simulink model "CM690A_HwAg0Meas"  (R2013b)
settings: Solver=FixedStepDiscrete  SolverMode=SingleTasking  StartTime=0.0  StopTime=22  FixedStep=0.002  RelTol=1e-3
undefined symbols (not defined in the file): ELECGLBPRM_DEGPERREV_DEGPERREV_F32, ELECGLBPRM_HWAGCENTROFFS_HWDEG_F32, ELECGLBPRM_HWAGSATNLOWRLIM_HWDEG_F32, ELECGLBPRM_HWAGSATNUPPRLIM_HWDEG_F32, ELECGLBPRM_HWAGSCA_ULS_F32, ELECGLBPRM_HWAGSPURGEARRAT_ULS_F32, ELECGLBPRM_HWAGSPURTORINGGEARRATSNSR0_ULS_F32, ELECGLBPRM_HWAGSPURTORINGGEARRATSNSR1_ULS_F32, ELECGLBPRM_NOFLT_CNT_U08, ELECGLBPRM_OFFSTRIMNOTPRFMD_CNT_U08, ELECGLBPRM_PRTCLFLT_CNT_U08, ELECGLBPRM_SKIPSTEPFLT_CNT_U08, ELECGLBPRM_SNSRINTFLT_CNT_U08, ELECGLBPRM_VRNRERRFLT_CNT_U08, FLTINJ_HWAG0MEAS_HWAG0, FLTINJ_HWAG0MEAS_TESTOK, HwAg0IfFlt, HwAg0MeasHwAg0IfFltFailStep, HwAg0MeasHwAg0IfFltPassStep, HwAg0MeasHwAg0Snsr0PrtclFltFailStep, HwAg0MeasHwAg0Snsr0PrtclFltPassStep, HwAg0MeasHwAg0Snsr1PrtclFltFailStep, HwAg0MeasHwAg0Snsr1PrtclFltPassStep, HwAg0MeasSnsr0Rev, HwAg0MeasSnsr1Rev, HwAg0MeasStep, HwAg0MeasVrnrErrThd, HwAg0MfgFlt, HwAg0Snsr0PrtclFlt, HwAg0Snsr1PrtclFlt, HWAG10THTOOTHTRIG_CNT_U08, HWAG11THTOOTHTRIG_CNT_U08, NtcSts1, sigbuilder_block, SigQlfr1
libraries: simulink x30, NxtrNvM x3
(part 3 of 5)

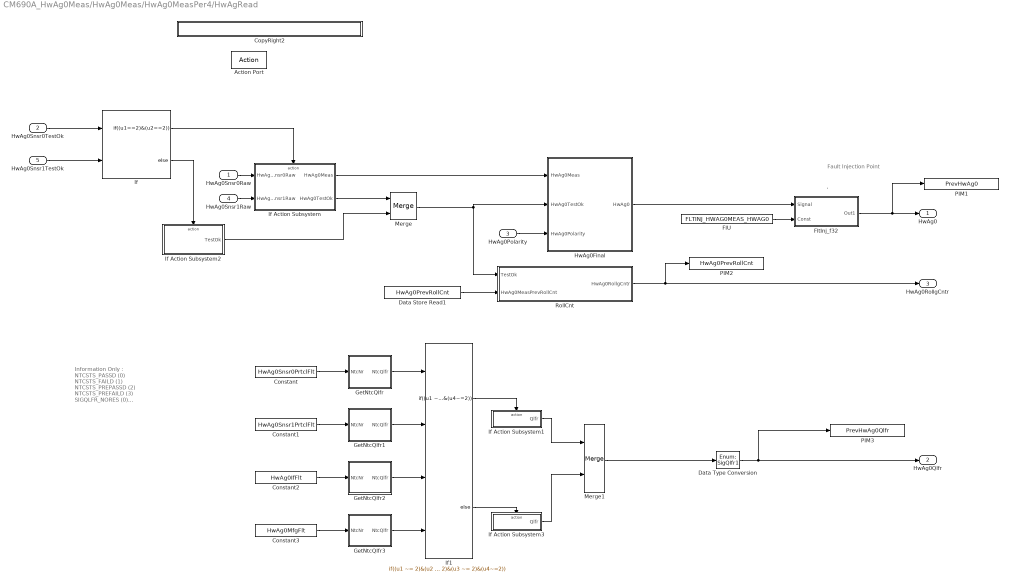
== system CM690A_HwAg0Meas/HwAg0Meas/HwAg0MeasPer4/HwAgRead ==
  note: ,
  note: Fault
      | Injection
      | Point
  note: Information Only :
      |
      | NTCSTS_PASSD            (0)
      | NTCSTS_FAILD              (1)
      | NTCSTS_PREPASSD    (2)
      | NTCSTS_PREFAILD      (3)
      |
      | SIGQLFR_NORES         (0)
      | SIGQLFR_PASSD          (1)
      | SIGQLFR_FAILD            (2)
  HwAg0Snsr0Raw : Inport
  HwAg0Snsr0TestOk : Inport  Port=2
  HwAg0Polarity : Inport  Port=3
  HwAg0Snsr1Raw : Inport  Port=4
  HwAg0Snsr1TestOk : Inport  Port=5
  Action Port : ActionPort  ActionType=then
  Constant : Constant  Value=HwAg0Snsr0PrtclFlt
  Constant1 : Constant  Value=HwAg0Snsr1PrtclFlt
  Constant2 : Constant  Value=HwAg0IfFlt
  Constant3 : Constant  Value=HwAg0MfgFlt
  CopyRight2 : Subsystem  Description=|  mask(Copyright Information){none=on}
      | Copyright info block.                                               
      |                                                                     
      | Place copyright information at the top of every subsystem in design.
      mask prompts: none "No parameters"
      mask help: Place copyright information at the top of every subsystem in design.
      mask Display:
      | NxtrConf = 'Nexteer Confidential';
      | 
      | sys = bdroot; %handle for the current model ("system")
      | first = get_param(sys,'Created');
      | first = first(end-3:end);  %year is last four digits
      | 
      | last = get_param(sys,'LastModifiedDate');
      | if isempty(last)
      |     last = datestr(now,'yyyy');
      | else
      |     last = last(end-3:end);
      | end
      | 
      | if strcmp(first,last)
      |     fprintf('%s -- Copyright %s Nexteer',NxtrConf,first)
      | else
      |     fprintf('%s -- %s%s- %s Nexteer',NxtrConf,char(169),first,last)
      | end
  Data Store Read1 : DataStoreRead  Priority=1  DataStoreName=HwAg0PrevRollCnt
  Data Type Conversion : DataTypeConversion  OutDataTypeStr=Enum: SigQlfr1
  FIU : Constant  Value=FLTINJ_HWAG0MEAS_HWAG0
  FltInj_f32 : Subsystem  RequirementInfo={'linktype_rmi_doors' '0000cf45 (/ESG Group/FDD Module Requirements/EA4 Specific/CM690A_HwAg0Meas)' '#CM690A_108' 'true' 'REQ: CM690A_108' '' } %GIDa_4c7341c4_5f9b_4469_826e_d49718259e6f  TreatAsAtomicUnit=on  VariantControl=FltInj_sim  mask(Fault_Injection){}
      mask help: Fault Injection is a simulation only block for EA4 programs.
  GetNtcQlfr : Subsystem
  GetNtcQlfr1 : Subsystem
  GetNtcQlfr2 : Subsystem
  GetNtcQlfr3 : Subsystem
  HwAg0Final : Subsystem  RequirementInfo={'linktype_rmi_doors' '0000cf45 (/ESG Group/FDD Module Requirements/EA4 Specific/CM690A_HwAg0Meas)' '#CM690A_29' 'true' 'REQ: CM690A_29' '' ; 'linktype_rmi_doors' '0000cf45 (/ESG Group/FDD Module Requirements/EA4 Specific/CM690A_HwAg0Meas)' '#CM690A_32' 'true' 'REQ: CM690A_32' '' ; 'linktype_rmi_doors' '0000cf45 (/ESG Group/FDD Module Requirements/EA4 Specific/CM690A_HwAg0Meas)' '#CM690A_90' 'true' 'REQ: CM690A_90' '' } %GIDa_315d8f1c_91b9_4fec_a381_d34b41dbf245
  If : If  NumInputs=2  IfExpression=(u1==2)&(u2==2)
  If Action Subsystem : Subsystem  TreatAsAtomicUnit=on
  If Action Subsystem1 : Subsystem  TreatAsAtomicUnit=on
  If Action Subsystem2 : Subsystem  TreatAsAtomicUnit=on
  If Action Subsystem3 : Subsystem  TreatAsAtomicUnit=on
  If1 : If  NumInputs=4  IfExpression=(u1 ~= 2)&(u2 ~= 2)&(u3 ~= 2)&(u4~=2)
  Merge : Merge
  Merge1 : Merge
  PIM1 : DataStoreWrite  RequirementInfo={} %GIDa_7b13e776_dea3_4ebd_98b9_3f5e270c50cd  DataStoreName=PrevHwAg0
  PIM2 : DataStoreWrite  RequirementInfo={} %GIDa_14d01694_55be_423b_b81c_a96afe431c02  Priority=2  DataStoreName=HwAg0PrevRollCnt
  PIM3 : DataStoreWrite  RequirementInfo={} %GIDa_a397fdff_e940_40b8_a32d_07bc645247b1  DataStoreName=PrevHwAg0Qlfr
  RollCnt : Stateflow chart  RequirementInfo={} %GIDa_138d63e5_0c8d_44c8_ba68_33eae6500659  TreatAsAtomicUnit=on
  HwAg0 : Outport  RequirementInfo={} %GIDa_98a3716a_95c6_4156_9aa9_7e286709311d
  HwAg0Qlfr : Outport  RequirementInfo={'linktype_rmi_doors' '0000cf45 (/ESG Group/FDD Module Requirements/EA4 Specific/CM690A_HwAg0Meas)' '#CM690A_30' 'true' 'REQ: CM690A_30' '' } %GIDa_8f926389_c076_467c_b7b7_a19e92fafcbc  Port=2
  HwAg0RollgCntr : Outport  RequirementInfo={'linktype_rmi_doors' '0000cf45 (/ESG Group/FDD Module Requirements/EA4 Specific/CM690A_HwAg0Meas)' '#CM690A_31' 'true' 'REQ: CM690A_31' '' } %GIDa_34151e8b_a860_45cc_acf4_67ec6eaad315  Port=3
  wires:
  RollCnt/1(HwAg0RollgCntr) -> PIM2/1, HwAg0RollgCntr/1
  Constant/1 -> GetNtcQlfr/1(NtcNr)
  HwAg0Snsr0TestOk/1 -> If/1
  HwAg0Snsr1TestOk/1 -> If/2
  If/1 -> If Action Subsystem/Action
  If/2 -> If Action Subsystem2/Action
  If Action Subsystem2/1(TestOk) -> Merge/2
  If Action Subsystem/1(HwAg0Meas) -> HwAg0Final/1(HwAg0Meas)
  HwAg0Final/1(HwAg0) -> FltInj_f32/1(Signal)
  Constant1/1 -> GetNtcQlfr1/1(NtcNr)
  Constant2/1 -> GetNtcQlfr2/1(NtcNr)
  GetNtcQlfr/1(NtcQlfr) -> If1/1
  GetNtcQlfr1/1(NtcQlfr) -> If1/2
  GetNtcQlfr2/1(NtcQlfr) -> If1/3
  If1/1 -> If Action Subsystem1/Action
  If1/2 -> If Action Subsystem3/Action
  If Action Subsystem1/1(Qlfr) -> Merge1/1
  If Action Subsystem3/1(Qlfr) -> Merge1/2
  If Action Subsystem/2(HwAg0TestOk) -> Merge/1
  HwAg0Polarity/1 -> HwAg0Final/3(HwAg0Polarity)
  GetNtcQlfr3/1(NtcQlfr) -> If1/4
  Constant3/1 -> GetNtcQlfr3/1(NtcNr)
  FIU/1 -> FltInj_f32/2(Const)
  Merge/1 -> HwAg0Final/2(HwAg0TestOk), RollCnt/1(TestOk)
  FltInj_f32/1(Out1) -> PIM1/1, HwAg0/1
  HwAg0Snsr0Raw/1 -> If Action Subsystem/1(HwAg0Snsr0Raw)
  HwAg0Snsr1Raw/1 -> If Action Subsystem/2(HwAg0Snsr1Raw)
  Data Store Read1/1 -> RollCnt/2(HwAg0MeasPrevRollCnt)
  Merge1/1 -> Data Type Conversion/1
  Data Type Conversion/1 -> PIM3/1, HwAg0Qlfr/1

== system CM690A_HwAg0Meas/HwAg0Meas/HwAg0MeasPer5/CopyRight2 ==

== system CM690A_HwAg0Meas/HwAg0Meas/HwAg0MeasPer5/If Action Subsystem ==
  Action Port : ActionPort  ActionType=then
  CopyRight2 : Subsystem  Description=|  mask(Copyright Information){none=on}
      | Copyright info block.                                               
      |                                                                     
      | Place copyright information at the top of every subsystem in design.
      mask prompts: none "No parameters"
      mask help: Place copyright information at the top of every subsystem in design.
      mask Display:
      | NxtrConf = 'Nexteer Confidential';
      | 
      | sys = bdroot; %handle for the current model ("system")
      | first = get_param(sys,'Created');
      | first = first(end-3:end);  %year is last four digits
      | 
      | last = get_param(sys,'LastModifiedDate');
      | if isempty(last)
      |     last = datestr(now,'yyyy');
      | else
      |     last = last(end-3:end);
      | end
      | 
      | if strcmp(first,last)
      |     fprintf('%s -- Copyright %s Nexteer',NxtrConf,first)
      | else
      |     fprintf('%s -- %s%s- %s Nexteer',NxtrConf,char(169),first,last)
      | end
  Data Type Conversion : DataTypeConversion  OutDataTypeStr=uint8
  NoFlt : Constant  RequirementInfo={} %GIDa_af25b43f_e757_49bd_94aa_be1229c5c8b6  Value=ELECGLBPRM_NOFLT_CNT_U08  OutDataTypeStr=uint8
  NtcSts : simulink/Sources/Enumerated Constant  OutDataTypeStr=Enum: NtcSts1  Value=NtcSts1.NTCSTS_PASSD  SampleTime=inf
  ParamByte : Outport
  TestOk : Outport  Port=2
  wires:
  NtcSts/1 -> Data Type Conversion/1
  NoFlt/1 -> ParamByte/1
  Data Type Conversion/1 -> TestOk/1

== system CM690A_HwAg0Meas/HwAg0Meas/HwAg0MeasPer5/If Action Subsystem1 ==
  Action Port : ActionPort  ActionType=else
  CopyRight2 : Subsystem  Description=|  mask(Copyright Information){none=on}
      | Copyright info block.                                               
      |                                                                     
      | Place copyright information at the top of every subsystem in design.
      mask prompts: none "No parameters"
      mask help: Place copyright information at the top of every subsystem in design.
      mask Display:
      | NxtrConf = 'Nexteer Confidential';
      | 
      | sys = bdroot; %handle for the current model ("system")
      | first = get_param(sys,'Created');
      | first = first(end-3:end);  %year is last four digits
      | 
      | last = get_param(sys,'LastModifiedDate');
      | if isempty(last)
      |     last = datestr(now,'yyyy');
      | else
      |     last = last(end-3:end);
      | end
      | 
      | if strcmp(first,last)
      |     fprintf('%s -- Copyright %s Nexteer',NxtrConf,first)
      | else
      |     fprintf('%s -- %s%s- %s Nexteer',NxtrConf,char(169),first,last)
      | end
  Data Type Conversion : DataTypeConversion  OutDataTypeStr=uint8
  NoFlt : Constant  RequirementInfo={} %GIDa_a79c1974_b7e9_4639_b05c_c7a17ce1d256  Value=ELECGLBPRM_OFFSTRIMNOTPRFMD_CNT_U08  OutDataTypeStr=uint8
  NtcSts : simulink/Sources/Enumerated Constant  OutDataTypeStr=Enum: NtcSts1  Value=NtcSts1.NTCSTS_FAILD  SampleTime=inf
  ParamByte : Outport
  TestOk : Outport  Port=2
  wires:
  NoFlt/1 -> ParamByte/1
  NtcSts/1 -> Data Type Conversion/1
  Data Type Conversion/1 -> TestOk/1

== system CM690A_HwAg0Meas/HwAg0Meas/HwAg0MeasPer5/SetNtcSts ==
  note: Note:
      |
      | - "ISO Fault Debounce Design" Simulink block intent to use here for Simulation purpose only. Do not Code this block
  NtcNr : Inport
  NtcStInfo : Inport  Port=2
  NtcSts : Inport  Port=3
  DebStep : Inport  Port=4
  CopyRight2 : Subsystem  Description=|  mask(Copyright Information){none=on}
      | Copyright info block.                                               
      |                                                                     
      | Place copyright information at the top of every subsystem in design.
      mask prompts: none "No parameters"
      mask help: Place copyright information at the top of every subsystem in design.
      mask Display:
      | NxtrConf = 'Nexteer Confidential';
      | 
      | sys = bdroot; %handle for the current model ("system")
      | first = get_param(sys,'Created');
      | first = first(end-3:end);  %year is last four digits
      | 
      | last = get_param(sys,'LastModifiedDate');
      | if isempty(last)
      |     last = datestr(now,'yyyy');
      | else
      |     last = last(end-3:end);
      | end
      | 
      | if strcmp(first,last)
      |     fprintf('%s -- Copyright %s Nexteer',NxtrConf,first)
      | else
      |     fprintf('%s -- %s%s- %s Nexteer',NxtrConf,char(169),first,last)
      | end
  Data Store Write : DataStoreWrite  DataStoreName=Ntc0X1F9Qlfr
  Ground : Ground
  ISO Fault Debounce Design : Stateflow chart  TreatAsAtomicUnit=on
      settings: AttributesFormatString=|
      | Simulation Purpose Only.
      | Do Not Code this block
      | Diagnostic Manager Owns this requirement
  Scope1 : Scope  NumInputPorts=3
      settings: YMin=-5~-5~-5  YMax=5~5~5  SaveName=ScopeData5
  Terminator : Terminator
  Terminator1 : Terminator
  wires:
  Ground/1 -> ISO Fault Debounce Design/3(SvcClr)
  ISO Fault Debounce Design/1(Qualifier) -> Data Store Write/1, Scope1/3
  DebStep/1 -> Scope1/2, ISO Fault Debounce Design/2(DebStep)
  NtcSts/1 -> Scope1/1, ISO Fault Debounce Design/1(NtcSts)
  NtcNr/1 -> Terminator/1
  NtcStInfo/1 -> Terminator1/1

== system CM690A_HwAg0Meas/HwAg0Meas/HwAg0MeasInit1/GetRefTmr1MicroSec32bit/CopyRight2 ==

== system CM690A_HwAg0Meas/HwAg0Meas/HwAg0MeasInit1/GetTiSpan1MicroSec32bit/CopyRight2 ==

== system CM690A_HwAg0Meas/HwAg0Meas/HwAg0MeasInit1/IoHwAb_SetFctPrphlHwAg0/CopyRight2 ==

== system CM690A_HwAg0Meas/HwAg0Meas/HwAg0MeasPer1/GetRefTmr1MicroSec32bit1/CopyRight2 ==

== system CM690A_HwAg0Meas/HwAg0Meas/HwAg0MeasPer1/GetTiSpan1MicroSec32bit/CopyRight2 ==

== system CM690A_HwAg0Meas/HwAg0Meas/HwAg0MeasPer1/IncrementCount/CopyRight2 ==

== system CM690A_HwAg0Meas/HwAg0Meas/HwAg0MeasPer1/ResetCount/CopyRight2 ==

== system CM690A_HwAg0Meas/HwAg0Meas/HwAg0MeasPer2/Snsr0Read/CopyRight2 ==

== system CM690A_HwAg0Meas/HwAg0Meas/HwAg0MeasPer2/Snsr0Read/DebStepSelection ==
  TestOk : Inport
  CopyRight2 : Subsystem  Description=|  mask(Copyright Information){none=on}
      | Copyright info block.                                               
      |                                                                     
      | Place copyright information at the top of every subsystem in design.
      mask prompts: none "No parameters"
      mask help: Place copyright information at the top of every subsystem in design.
      mask Display:
      | NxtrConf = 'Nexteer Confidential';
      | 
      | sys = bdroot; %handle for the current model ("system")
      | first = get_param(sys,'Created');
      | first = first(end-3:end);  %year is last four digits
      | 
      | last = get_param(sys,'LastModifiedDate');
      | if isempty(last)
      |     last = datestr(now,'yyyy');
      | else
      |     last = last(end-3:end);
      | end
      | 
      | if strcmp(first,last)
      |     fprintf('%s -- Copyright %s Nexteer',NxtrConf,first)
      | else
      |     fprintf('%s -- %s%s- %s Nexteer',NxtrConf,char(169),first,last)
      | end
  NTCFailStepCal : Constant  Value=HwAg0MeasHwAg0Snsr0PrtclFltFailStep
  NTCPassStepCal : Constant  Value=HwAg0MeasHwAg0Snsr0PrtclFltPassStep
  Switch : Switch  Criteria=u2 > Threshold  Threshold=2
  DebStep : Outport  OutDataTypeStr=uint16
  wires:
  NTCFailStepCal/1 -> Switch/1
  Switch/1 -> DebStep/1
  NTCPassStepCal/1 -> Switch/3
  TestOk/1 -> Switch/2

== system CM690A_HwAg0Meas/HwAg0Meas/HwAg0MeasPer2/Snsr0Read/Do nothing ==
  Action Port : ActionPort  ActionType=else
  CopyRight2 : Subsystem  Description=|  mask(Copyright Information){none=on}
      | Copyright info block.                                               
      |                                                                     
      | Place copyright information at the top of every subsystem in design.
      mask prompts: none "No parameters"
      mask help: Place copyright information at the top of every subsystem in design.
      mask Display:
      | NxtrConf = 'Nexteer Confidential';
      | 
      | sys = bdroot; %handle for the current model ("system")
      | first = get_param(sys,'Created');
      | first = first(end-3:end);  %year is last four digits
      | 
      | last = get_param(sys,'LastModifiedDate');
      | if isempty(last)
      |     last = datestr(now,'yyyy');
      | else
      |     last = last(end-3:end);
      | end
      | 
      | if strcmp(first,last)
      |     fprintf('%s -- Copyright %s Nexteer',NxtrConf,first)
      | else
      |     fprintf('%s -- %s%s- %s Nexteer',NxtrConf,char(169),first,last)
      | end

== system CM690A_HwAg0Meas/HwAg0Meas/HwAg0MeasPer2/Snsr0Read/RawHwAgRead ==
  Snsr0CS : Inport
  Snsr0FRS : Inport  Port=2
  Snsr0FCCN : Inport  Port=3
  Snsr0Data : Inport  Port=4
  Snsr0Id : Inport  Port=5
  Bus Selector : BusSelector  OutputSignals=RawHwAg,TestOk,ParamByte
  Bus Selector1 : BusSelector  OutputSignals=RawHwAg,TestOk,ParamByte
  CopyRight2 : Subsystem  Description=|  mask(Copyright Information){none=on}
      | Copyright info block.                                               
      |                                                                     
      | Place copyright information at the top of every subsystem in design.
      mask prompts: none "No parameters"
      mask help: Place copyright information at the top of every subsystem in design.
      mask Display:
      | NxtrConf = 'Nexteer Confidential';
      | 
      | sys = bdroot; %handle for the current model ("system")
      | first = get_param(sys,'Created');
      | first = first(end-3:end);  %year is last four digits
      | 
      | last = get_param(sys,'LastModifiedDate');
      | if isempty(last)
      |     last = datestr(now,'yyyy');
      | else
      |     last = last(end-3:end);
      | end
      | 
      | if strcmp(first,last)
      |     fprintf('%s -- Copyright %s Nexteer',NxtrConf,first)
      | else
      |     fprintf('%s -- %s%s- %s Nexteer',NxtrConf,char(169),first,last)
      | end
  If : If  RequirementInfo={} %GIDa_46781e8b_8ae4_49ab_b4ce_f2a8b4411ed9  IfExpression=u1 ~= 0
  Merge : Merge
  Merge1 : Merge
  Merge2 : Merge
  NewMsg : Subsystem  TreatAsAtomicUnit=on
  NoNewMsg : Subsystem  RequirementInfo={'linktype_rmi_doors' '0000cf45 (/ESG Group/FDD Module Requirements/EA4 Specific/CM690A_HwAg0Meas)' '#CM690A_47' 'true' 'REQ: CM690A_47' '' } %GIDa_ed38ddaf_6377_4824_8afe_3c38153c265e  TreatAsAtomicUnit=on
      mask Display: disp('NoNewMsg')
  RawHwAg : Outport
  TestOk : Outport  Port=2
  ParamByte : Outport  Port=3
  wires:
  Snsr0FRS/1 -> If/1
  If/1 -> NewMsg/Action  "NoFault"
  If/2 -> NoNewMsg/Action  "Fault"
  Snsr0CS/1 -> NewMsg/1(Snsr0CS)
  NewMsg/1(Out1) -> Bus Selector/1
  NoNewMsg/1(Out1) -> Bus Selector1/1
  Bus Selector1/1 -> Merge2/1  "<RawHwAg>"
  Bus Selector/1 -> Merge2/2  "<RawHwAg>"
  Bus Selector1/2 -> Merge/1  "<TestOk>"
  Bus Selector/2 -> Merge/2  "<TestOk>"
  Bus Selector1/3 -> Merge1/1  "<ParamByte>"
  Bus Selector/3 -> Merge1/2  "<ParamByte>"
  Merge2/1 -> RawHwAg/1  "RawHwAg"
  Merge/1 -> TestOk/1  "TestOk"
  Merge1/1 -> ParamByte/1  "ParamByte"
  Snsr0FCCN/1 -> NewMsg/2(Snsr0FCCN)
  Snsr0Data/1 -> NewMsg/4(Snsr0Data)
  Snsr0Id/1 -> NewMsg/3(Snsr0Id)

== system CM690A_HwAg0Meas/HwAg0Meas/HwAg0MeasPer2/Snsr0Read/Read the Flag ==
  RegInpRSENT4FND : Inport
  Action Port : ActionPort  ActionType=then
  CopyRight2 : Subsystem  Description=|  mask(Copyright Information){none=on}
      | Copyright info block.                                               
      |                                                                     
      | Place copyright information at the top of every subsystem in design.
      mask prompts: none "No parameters"
      mask help: Place copyright information at the top of every subsystem in design.
      mask Display:
      | NxtrConf = 'Nexteer Confidential';
      | 
      | sys = bdroot; %handle for the current model ("system")
      | first = get_param(sys,'Created');
      | first = first(end-3:end);  %year is last four digits
      | 
      | last = get_param(sys,'LastModifiedDate');
      | if isempty(last)
      |     last = datestr(now,'yyyy');
      | else
      |     last = last(end-3:end);
      | end
      | 
      | if strcmp(first,last)
      |     fprintf('%s -- Copyright %s Nexteer',NxtrConf,first)
      | else
      |     fprintf('%s -- %s%s- %s Nexteer',NxtrConf,char(169),first,last)
      | end
  RSENT4DummyRead : Terminator
  wires:
  RegInpRSENT4FND/1 -> RSENT4DummyRead/1

== system CM690A_HwAg0Meas/HwAg0Meas/HwAg0MeasPer2/Snsr0Read/SetNtcSts ==
  note: Note:
      |
      | - "ISO Fault Debounce Design" Simulink block intent to use here for Simulation purpose only. Do not Code this block
  NtcNr : Inport
  NtcStInfo : Inport  Port=2
  NtcSts : Inport  Port=3
  DebStep : Inport  Port=4
  CopyRight2 : Subsystem  Description=|  mask(Copyright Information){none=on}
      | Copyright info block.                                               
      |                                                                     
      | Place copyright information at the top of every subsystem in design.
      mask prompts: none "No parameters"
      mask help: Place copyright information at the top of every subsystem in design.
      mask Display:
      | NxtrConf = 'Nexteer Confidential';
      | 
      | sys = bdroot; %handle for the current model ("system")
      | first = get_param(sys,'Created');
      | first = first(end-3:end);  %year is last four digits
      | 
      | last = get_param(sys,'LastModifiedDate');
      | if isempty(last)
      |     last = datestr(now,'yyyy');
      | else
      |     last = last(end-3:end);
      | end
      | 
      | if strcmp(first,last)
      |     fprintf('%s -- Copyright %s Nexteer',NxtrConf,first)
      | else
      |     fprintf('%s -- %s%s- %s Nexteer',NxtrConf,char(169),first,last)
      | end
  Data Store Write : DataStoreWrite  DataStoreName=Ntc0x093Qlfr
  Ground : Ground
  ISO Fault Debounce Design : Stateflow chart  TreatAsAtomicUnit=on
      settings: AttributesFormatString=|
      | Simulation Purpose Only.
      | Do Not Code this block
      | Diagnostic Manager Owns this requirement
  Scope1 : Scope  NumInputPorts=3
      settings: YMin=-5~-5~-5  YMax=5~5~5  SaveName=ScopeData5
  Terminator : Terminator
  Terminator1 : Terminator
  wires:
  Ground/1 -> ISO Fault Debounce Design/3(SvcClr)
  ISO Fault Debounce Design/1(Qualifier) -> Data Store Write/1, Scope1/3
  DebStep/1 -> Scope1/2, ISO Fault Debounce Design/2(DebStep)
  NtcSts/1 -> Scope1/1, ISO Fault Debounce Design/1(NtcSts)
  NtcNr/1 -> Terminator/1
  NtcStInfo/1 -> Terminator1/1

== system CM690A_HwAg0Meas/HwAg0Meas/HwAg0MeasPer2/Snsr0Read1/CopyRight2 ==

== system CM690A_HwAg0Meas/HwAg0Meas/HwAg0MeasPer3/Snsr1Read/CopyRight2 ==

== system CM690A_HwAg0Meas/HwAg0Meas/HwAg0MeasPer3/Snsr1Read/DebStepSelection ==
  TestOk : Inport
  CopyRight2 : Subsystem  Description=|  mask(Copyright Information){none=on}
      | Copyright info block.                                               
      |                                                                     
      | Place copyright information at the top of every subsystem in design.
      mask prompts: none "No parameters"
      mask help: Place copyright information at the top of every subsystem in design.
      mask Display:
      | NxtrConf = 'Nexteer Confidential';
      | 
      | sys = bdroot; %handle for the current model ("system")
      | first = get_param(sys,'Created');
      | first = first(end-3:end);  %year is last four digits
      | 
      | last = get_param(sys,'LastModifiedDate');
      | if isempty(last)
      |     last = datestr(now,'yyyy');
      | else
      |     last = last(end-3:end);
      | end
      | 
      | if strcmp(first,last)
      |     fprintf('%s -- Copyright %s Nexteer',NxtrConf,first)
      | else
      |     fprintf('%s -- %s%s- %s Nexteer',NxtrConf,char(169),first,last)
      | end
  NTCFailStepCal : Constant  Value=HwAg0MeasHwAg0Snsr1PrtclFltFailStep
  NTCPassStepCal : Constant  Value=HwAg0MeasHwAg0Snsr1PrtclFltPassStep
  Switch : Switch  Criteria=u2 > Threshold  Threshold=2
  DebStep : Outport  OutDataTypeStr=uint16
  wires:
  NTCFailStepCal/1 -> Switch/1
  Switch/1 -> DebStep/1
  NTCPassStepCal/1 -> Switch/3
  TestOk/1 -> Switch/2

== system CM690A_HwAg0Meas/HwAg0Meas/HwAg0MeasPer3/Snsr1Read/Do nothing1 ==
  Action Port : ActionPort  ActionType=else
  CopyRight2 : Subsystem  Description=|  mask(Copyright Information){none=on}
      | Copyright info block.                                               
      |                                                                     
      | Place copyright information at the top of every subsystem in design.
      mask prompts: none "No parameters"
      mask help: Place copyright information at the top of every subsystem in design.
      mask Display:
      | NxtrConf = 'Nexteer Confidential';
      | 
      | sys = bdroot; %handle for the current model ("system")
      | first = get_param(sys,'Created');
      | first = first(end-3:end);  %year is last four digits
      | 
      | last = get_param(sys,'LastModifiedDate');
      | if isempty(last)
      |     last = datestr(now,'yyyy');
      | else
      |     last = last(end-3:end);
      | end
      | 
      | if strcmp(first,last)
      |     fprintf('%s -- Copyright %s Nexteer',NxtrConf,first)
      | else
      |     fprintf('%s -- %s%s- %s Nexteer',NxtrConf,char(169),first,last)
      | end

== system CM690A_HwAg0Meas/HwAg0Meas/HwAg0MeasPer3/Snsr1Read/Do nothing2 ==
  Action Port : ActionPort  ActionType=else
  CopyRight2 : Subsystem  Description=|  mask(Copyright Information){none=on}
      | Copyright info block.                                               
      |                                                                     
      | Place copyright information at the top of every subsystem in design.
      mask prompts: none "No parameters"
      mask help: Place copyright information at the top of every subsystem in design.
      mask Display:
      | NxtrConf = 'Nexteer Confidential';
      | 
      | sys = bdroot; %handle for the current model ("system")
      | first = get_param(sys,'Created');
      | first = first(end-3:end);  %year is last four digits
      | 
      | last = get_param(sys,'LastModifiedDate');
      | if isempty(last)
      |     last = datestr(now,'yyyy');
      | else
      |     last = last(end-3:end);
      | end
      | 
      | if strcmp(first,last)
      |     fprintf('%s -- Copyright %s Nexteer',NxtrConf,first)
      | else
      |     fprintf('%s -- %s%s- %s Nexteer',NxtrConf,char(169),first,last)
      | end

== system CM690A_HwAg0Meas/HwAg0Meas/HwAg0MeasPer3/Snsr1Read/RawHwAgRead ==
  Snsr1CS : Inport
  Snsr1FRS : Inport  Port=2
  Snsr1FCCN : Inport  Port=3
  Snsr1Data : Inport  Port=4
  Snsr1Id : Inport  Port=5
  Bus Selector : BusSelector  OutputSignals=RawHwAg,TestOk,ParamByte
  Bus Selector1 : BusSelector  OutputSignals=RawHwAg,TestOk,ParamByte
  CopyRight2 : Subsystem  Description=|  mask(Copyright Information){none=on}
      | Copyright info block.                                               
      |                                                                     
      | Place copyright information at the top of every subsystem in design.
      mask prompts: none "No parameters"
      mask help: Place copyright information at the top of every subsystem in design.
      mask Display:
      | NxtrConf = 'Nexteer Confidential';
      | 
      | sys = bdroot; %handle for the current model ("system")
      | first = get_param(sys,'Created');
      | first = first(end-3:end);  %year is last four digits
      | 
      | last = get_param(sys,'LastModifiedDate');
      | if isempty(last)
      |     last = datestr(now,'yyyy');
      | else
      |     last = last(end-3:end);
      | end
      | 
      | if strcmp(first,last)
      |     fprintf('%s -- Copyright %s Nexteer',NxtrConf,first)
      | else
      |     fprintf('%s -- %s%s- %s Nexteer',NxtrConf,char(169),first,last)
      | end
  If : If  RequirementInfo={} %GIDa_7644cdbb_66a8_49f6_a4d4_60348c8cfce1  IfExpression=u1 ~= 0
  Merge : Merge
  Merge1 : Merge
  Merge2 : Merge
  NewMsg : Subsystem  TreatAsAtomicUnit=on
  NoNewMsg : Subsystem  RequirementInfo={'linktype_rmi_doors' '0000cf45 (/ESG Group/FDD Module Requirements/EA4 Specific/CM690A_HwAg0Meas)' '#CM690A_64' 'true' 'REQ: CM690A_64' '' } %GIDa_10b4e8f5_e554_4d89_a490_9a22ba77e950  TreatAsAtomicUnit=on
      mask Display: disp('NoNewMsg')
  RawHwAg : Outport
  TestOk : Outport  Port=2
  ParamByte : Outport  Port=3
  wires:
  Snsr1FRS/1 -> If/1
  If/1 -> NewMsg/Action  "NoFault"
  If/2 -> NoNewMsg/Action  "Fault"
  Snsr1CS/1 -> NewMsg/1(Snsr1CS)
  NewMsg/1(Out1) -> Bus Selector/1
  NoNewMsg/1(Out1) -> Bus Selector1/1
  Bus Selector1/1 -> Merge2/1  "<RawHwAg>"
  Bus Selector/1 -> Merge2/2  "<RawHwAg>"
  Bus Selector1/2 -> Merge/1  "<TestOk>"
  Bus Selector/2 -> Merge/2  "<TestOk>"
  Bus Selector1/3 -> Merge1/1  "<ParamByte>"
  Bus Selector/3 -> Merge1/2  "<ParamByte>"
  Merge2/1 -> RawHwAg/1  "RawHwAg"
  Merge/1 -> TestOk/1  "TestOk"
  Merge1/1 -> ParamByte/1  "ParamByte"
  Snsr1FCCN/1 -> NewMsg/2(Snsr1FCCN)
  Snsr1Data/1 -> NewMsg/4(Snsr1Data)
  Snsr1Id/1 -> NewMsg/3(Snsr1Id)

== system CM690A_HwAg0Meas/HwAg0Meas/HwAg0MeasPer3/Snsr1Read/Read the Flag ==
  RegInpRSENT4FND : Inport
  Action Port : ActionPort  ActionType=then
  CopyRight2 : Subsystem  Description=|  mask(Copyright Information){none=on}
      | Copyright info block.                                               
      |                                                                     
      | Place copyright information at the top of every subsystem in design.
      mask prompts: none "No parameters"
      mask help: Place copyright information at the top of every subsystem in design.
      mask Display:
      | NxtrConf = 'Nexteer Confidential';
      | 
      | sys = bdroot; %handle for the current model ("system")
      | first = get_param(sys,'Created');
      | first = first(end-3:end);  %year is last four digits
      | 
      | last = get_param(sys,'LastModifiedDate');
      | if isempty(last)
      |     last = datestr(now,'yyyy');
      | else
      |     last = last(end-3:end);
      | end
      | 
      | if strcmp(first,last)
      |     fprintf('%s -- Copyright %s Nexteer',NxtrConf,first)
      | else
      |     fprintf('%s -- %s%s- %s Nexteer',NxtrConf,char(169),first,last)
      | end
  RSENT4DummyRead : Terminator
  wires:
  RegInpRSENT4FND/1 -> RSENT4DummyRead/1

== system CM690A_HwAg0Meas/HwAg0Meas/HwAg0MeasPer3/Snsr1Read/SetNtcSts ==
  note: Note:
      |
      | - "ISO Fault Debounce Design" Simulink block intent to use here for Simulation purpose only. Do not Code this block
  NtcNr : Inport
  NtcStInfo : Inport  Port=2
  NtcSts : Inport  Port=3
  DebStep : Inport  Port=4
  CopyRight2 : Subsystem  Description=|  mask(Copyright Information){none=on}
      | Copyright info block.                                               
      |                                                                     
      | Place copyright information at the top of every subsystem in design.
      mask prompts: none "No parameters"
      mask help: Place copyright information at the top of every subsystem in design.
      mask Display:
      | NxtrConf = 'Nexteer Confidential';
      | 
      | sys = bdroot; %handle for the current model ("system")
      | first = get_param(sys,'Created');
      | first = first(end-3:end);  %year is last four digits
      | 
      | last = get_param(sys,'LastModifiedDate');
      | if isempty(last)
      |     last = datestr(now,'yyyy');
      | else
      |     last = last(end-3:end);
      | end
      | 
      | if strcmp(first,last)
      |     fprintf('%s -- Copyright %s Nexteer',NxtrConf,first)
      | else
      |     fprintf('%s -- %s%s- %s Nexteer',NxtrConf,char(169),first,last)
      | end
  Data Store Write : DataStoreWrite  DataStoreName=Ntc0x095Qlfr
  Ground : Ground
  ISO Fault Debounce Design : Stateflow chart  TreatAsAtomicUnit=on
      settings: AttributesFormatString=|
      | Simulation Purpose Only.
      | Do Not Code this block
      | Diagnostic Manager Owns this requirement
  Scope1 : Scope  NumInputPorts=3
      settings: YMin=-5~-5~-5  YMax=5~5~5  SaveName=ScopeData5
  Terminator : Terminator
  Terminator1 : Terminator
  wires:
  Ground/1 -> ISO Fault Debounce Design/3(SvcClr)
  ISO Fault Debounce Design/1(Qualifier) -> Data Store Write/1, Scope1/3
  DebStep/1 -> Scope1/2, ISO Fault Debounce Design/2(DebStep)
  NtcSts/1 -> Scope1/1, ISO Fault Debounce Design/1(NtcSts)
  NtcNr/1 -> Terminator/1
  NtcStInfo/1 -> Terminator1/1

== system CM690A_HwAg0Meas/HwAg0Meas/HwAg0MeasPer3/Snsr1Read/SyncPulse ==
  note: Information only:
      |
      | - Sensors are synchronized if they receive 104us tick wide SPCT low pulse.
  note: Follow below steps in same order:
      |
      | 1. Send Sensor Synchronization command Pulse (RegOutRSENT4SPCT = 103U)
      | 1a. asm"syncm"
      | 2. NRS Flag Check: If the flag (RegInpRSENT4NRS==1) is Set Clear the flag RegOutRSENT4NRC=1
      | 2a. 2us wait timer
      | 3. Execute RegOutRSENT4SPCT = 103U
  RegInpRSENT4NRS : Inport
  Action Port : ActionPort  ActionType=then
  CopyRight2 : Subsystem  Description=|  mask(Copyright Information){none=on}
      | Copyright info block.                                               
      |                                                                     
      | Place copyright information at the top of every subsystem in design.
      mask prompts: none "No parameters"
      mask help: Place copyright information at the top of every subsystem in design.
      mask Display:
      | NxtrConf = 'Nexteer Confidential';
      | 
      | sys = bdroot; %handle for the current model ("system")
      | first = get_param(sys,'Created');
      | first = first(end-3:end);  %year is last four digits
      | 
      | last = get_param(sys,'LastModifiedDate');
      | if isempty(last)
      |     last = datestr(now,'yyyy');
      | else
      |     last = last(end-3:end);
      | end
      | 
      | if strcmp(first,last)
      |     fprintf('%s -- Copyright %s Nexteer',NxtrConf,first)
      | else
      |     fprintf('%s -- %s%s- %s Nexteer',NxtrConf,char(169),first,last)
      | end
  GetRefTmr1MicroSec32bit : Subsystem
      settings: AttributesFormatString=Client Call : Start Time
  GetTiSpan1MicroSec32bit : Subsystem
  Ground1 : Ground
  Ground2 : Ground
  Terminator : Terminator
  Terminator1 : Terminator
  RegOutRSENT4SPCT : Outport
  RegOutRSENT4NRC : Outport  Port=2
  wires:
  Ground1/1 -> RegOutRSENT4SPCT/1
  Ground2/1 -> RegOutRSENT4NRC/1
  RegInpRSENT4NRS/1 -> Terminator/1
  GetTiSpan1MicroSec32bit/1(TiSpan) -> Terminator1/1
  GetRefTmr1MicroSec32bit/1(RefTmr) -> GetTiSpan1MicroSec32bit/1(RefTmr)

== system CM690A_HwAg0Meas/HwAg0Meas/HwAg0MeasPer3/Snsr1Read1/CopyRight2 ==

== system CM690A_HwAg0Meas/HwAg0Meas/HwAg0MeasPer4/HwAgPrevRead/CopyRight2 ==

== system CM690A_HwAg0Meas/HwAg0Meas/HwAg0MeasPer4/HwAgRead/CopyRight2 ==

== system CM690A_HwAg0Meas/HwAg0Meas/HwAg0MeasPer4/HwAgRead/FltInj_f32 ==
  note: Inport #2 must be constant
      | Const: FltInjectionLocType
  note: EA4.x Fault Injection
  note: This block requires no modification by FDD author.
      |
      | This block does not actually simulate any fault injection.  It is simply a pass-thru.
      |
      | The Const port (#2) simply terminates its signal, but we are trying to force the FDD author
      | to properly use the FltInjectionLocType enumeration in FDD model.
  Signal : Inport
  Const : Inport  Port=2
  Terminator : Terminator
  Out1 : Outport
  wires:
  Const/1 -> Terminator/1
  Signal/1 -> Out1/1

== system CM690A_HwAg0Meas/HwAg0Meas/HwAg0MeasPer4/HwAgRead/GetNtcQlfr ==
  NtcNr : Inport
  CopyRight2 : Subsystem  Description=|  mask(Copyright Information){none=on}
      | Copyright info block.                                               
      |                                                                     
      | Place copyright information at the top of every subsystem in design.
      mask prompts: none "No parameters"
      mask help: Place copyright information at the top of every subsystem in design.
      mask Display:
      | NxtrConf = 'Nexteer Confidential';
      | 
      | sys = bdroot; %handle for the current model ("system")
      | first = get_param(sys,'Created');
      | first = first(end-3:end);  %year is last four digits
      | 
      | last = get_param(sys,'LastModifiedDate');
      | if isempty(last)
      |     last = datestr(now,'yyyy');
      | else
      |     last = last(end-3:end);
      | end
      | 
      | if strcmp(first,last)
      |     fprintf('%s -- Copyright %s Nexteer',NxtrConf,first)
      | else
      |     fprintf('%s -- %s%s- %s Nexteer',NxtrConf,char(169),first,last)
      | end
  Data Store Read : DataStoreRead  DataStoreName=Ntc0x093Qlfr
  Terminator : Terminator
  NtcQlfr : Outport
  wires:
  Data Store Read/1 -> NtcQlfr/1
  NtcNr/1 -> Terminator/1

== system CM690A_HwAg0Meas/HwAg0Meas/HwAg0MeasPer4/HwAgRead/GetNtcQlfr1 ==
  NtcNr : Inport
  CopyRight2 : Subsystem  Description=|  mask(Copyright Information){none=on}
      | Copyright info block.                                               
      |                                                                     
      | Place copyright information at the top of every subsystem in design.
      mask prompts: none "No parameters"
      mask help: Place copyright information at the top of every subsystem in design.
      mask Display:
      | NxtrConf = 'Nexteer Confidential';
      | 
      | sys = bdroot; %handle for the current model ("system")
      | first = get_param(sys,'Created');
      | first = first(end-3:end);  %year is last four digits
      | 
      | last = get_param(sys,'LastModifiedDate');
      | if isempty(last)
      |     last = datestr(now,'yyyy');
      | else
      |     last = last(end-3:end);
      | end
      | 
      | if strcmp(first,last)
      |     fprintf('%s -- Copyright %s Nexteer',NxtrConf,first)
      | else
      |     fprintf('%s -- %s%s- %s Nexteer',NxtrConf,char(169),first,last)
      | end
  Data Store Read : DataStoreRead  DataStoreName=Ntc0x095Qlfr
  Terminator : Terminator
  NtcQlfr : Outport
  wires:
  Data Store Read/1 -> NtcQlfr/1
  NtcNr/1 -> Terminator/1

== system CM690A_HwAg0Meas/HwAg0Meas/HwAg0MeasPer4/HwAgRead/GetNtcQlfr2 ==
  NtcNr : Inport
  CopyRight2 : Subsystem  Description=|  mask(Copyright Information){none=on}
      | Copyright info block.                                               
      |                                                                     
      | Place copyright information at the top of every subsystem in design.
      mask prompts: none "No parameters"
      mask help: Place copyright information at the top of every subsystem in design.
      mask Display:
      | NxtrConf = 'Nexteer Confidential';
      | 
      | sys = bdroot; %handle for the current model ("system")
      | first = get_param(sys,'Created');
      | first = first(end-3:end);  %year is last four digits
      | 
      | last = get_param(sys,'LastModifiedDate');
      | if isempty(last)
      |     last = datestr(now,'yyyy');
      | else
      |     last = last(end-3:end);
      | end
      | 
      | if strcmp(first,last)
      |     fprintf('%s -- Copyright %s Nexteer',NxtrConf,first)
      | else
      |     fprintf('%s -- %s%s- %s Nexteer',NxtrConf,char(169),first,last)
      | end
  Data Store Read : DataStoreRead  DataStoreName=Ntc0x094Qlfr
  Terminator : Terminator
  NtcQlfr : Outport
  wires:
  Data Store Read/1 -> NtcQlfr/1
  NtcNr/1 -> Terminator/1

== system CM690A_HwAg0Meas/HwAg0Meas/HwAg0MeasPer4/HwAgRead/GetNtcQlfr3 ==
  NtcNr : Inport
  CopyRight2 : Subsystem  Description=|  mask(Copyright Information){none=on}
      | Copyright info block.                                               
      |                                                                     
      | Place copyright information at the top of every subsystem in design.
      mask prompts: none "No parameters"
      mask help: Place copyright information at the top of every subsystem in design.
      mask Display:
      | NxtrConf = 'Nexteer Confidential';
      | 
      | sys = bdroot; %handle for the current model ("system")
      | first = get_param(sys,'Created');
      | first = first(end-3:end);  %year is last four digits
      | 
      | last = get_param(sys,'LastModifiedDate');
      | if isempty(last)
      |     last = datestr(now,'yyyy');
      | else
      |     last = last(end-3:end);
      | end
      | 
      | if strcmp(first,last)
      |     fprintf('%s -- Copyright %s Nexteer',NxtrConf,first)
      | else
      |     fprintf('%s -- %s%s- %s Nexteer',NxtrConf,char(169),first,last)
      | end
  Data Store Read : DataStoreRead  DataStoreName=Ntc0X1F9Qlfr
  Terminator : Terminator
  NtcQlfr : Outport
  wires:
  Data Store Read/1 -> NtcQlfr/1
  NtcNr/1 -> Terminator/1

== system CM690A_HwAg0Meas/HwAg0Meas/HwAg0MeasPer4/HwAgRead/HwAg0Final ==
  HwAg0Meas : Inport  OutDataTypeStr=single
  HwAg0TestOk : Inport  Port=2
  HwAg0Polarity : Inport  Port=3
  CopyRight2 : Subsystem  Description=|  mask(Copyright Information){none=on}
      | Copyright info block.                                               
      |                                                                     
      | Place copyright information at the top of every subsystem in design.
      mask prompts: none "No parameters"
      mask help: Place copyright information at the top of every subsystem in design.
      mask Display:
      | NxtrConf = 'Nexteer Confidential';
      | 
      | sys = bdroot; %handle for the current model ("system")
      | first = get_param(sys,'Created');
      | first = first(end-3:end);  %year is last four digits
      | 
      | last = get_param(sys,'LastModifiedDate');
      | if isempty(last)
      |     last = datestr(now,'yyyy');
      | else
      |     last = last(end-3:end);
      | end
      | 
      | if strcmp(first,last)
      |     fprintf('%s -- Copyright %s Nexteer',NxtrConf,first)
      | else
      |     fprintf('%s -- %s%s- %s Nexteer',NxtrConf,char(169),first,last)
      | end
  ModRoll : Stateflow chart  RequirementInfo={} %GIDa_b6f0793a_f36e_4f33_a919_cdec60db1678  TreatAsAtomicUnit=on
  NVM Shadow RAM : DataStoreRead  DataStoreName=HwAg0OffsTrim
  PIM : DataStoreWrite  RequirementInfo={'linktype_rmi_doors' '0000cf45 (/ESG Group/FDD Module Requirements/EA4 Specific/CM690A_HwAg0Meas)' '#CM690A_91' 'true' 'REQ: CM690A_91' '' } %GIDa_daebfb9a_41b6_403c_982a_2244515c0a47  DataStoreName=HwAg0PrevHwAg0
  PIM1 : DataStoreRead  DataStoreName=HwAg0PrevHwAg0
  Product : Product
  Saturation : Saturate  UpperLimit=ELECGLBPRM_HWAGSATNUPPRLIM_HWDEG_F32  LowerLimit=ELECGLBPRM_HWAGSATNLOWRLIM_HWDEG_F32
  Subtract1 : Sum  Inputs=+-
  Switch : Switch  Criteria=u2 > Threshold  Threshold=2
  HwAg0 : Outport  RequirementInfo={'linktype_rmi_doors' '0000cf45 (/ESG Group/FDD Module Requirements/EA4 Specific/CM690A_HwAg0Meas)' '#CM690A_26' 'true' 'REQ: CM690A_26' '' } %GIDa_584b7e1b_40b1_43ad_ab72_5fdceecef2f0
  wires:
  Product/1 -> Switch/3
  Switch/1 -> Subtract1/1, PIM/1
  HwAg0TestOk/1 -> Switch/2
  Subtract1/1 -> ModRoll/1(RawVal)
  HwAg0Meas/1 -> Product/1
  HwAg0Polarity/1 -> Product/2
  NVM Shadow RAM/1 -> Subtract1/2
  Saturation/1 -> HwAg0/1
  ModRoll/1(OutVal) -> Saturation/1
  PIM1/1 -> Switch/1

== system CM690A_HwAg0Meas/HwAg0Meas/HwAg0MeasPer4/HwAgRead/If Action Subsystem ==
  note: Information only:
      |
      | - AbsoluteHandWheel Angle Calculation
  HwAg0Snsr0Raw : Inport
  HwAg0Snsr1Raw : Inport  Port=2
  Action Port : ActionPort  PropagateVarSize=During execution  ActionType=then
  AdjStepCalc : Subsystem
  Constant : Constant  Value=HwAg0IfFlt
  CopyRight2 : Subsystem  Description=|  mask(Copyright Information){none=on}
      | Copyright info block.                                               
      |                                                                     
      | Place copyright information at the top of every subsystem in design.
      mask prompts: none "No parameters"
      mask help: Place copyright information at the top of every subsystem in design.
      mask Display:
      | NxtrConf = 'Nexteer Confidential';
      | 
      | sys = bdroot; %handle for the current model ("system")
      | first = get_param(sys,'Created');
      | first = first(end-3:end);  %year is last four digits
      | 
      | last = get_param(sys,'LastModifiedDate');
      | if isempty(last)
      |     last = datestr(now,'yyyy');
      | else
      |     last = last(end-3:end);
      | end
      | 
      | if strcmp(first,last)
      |     fprintf('%s -- Copyright %s Nexteer',NxtrConf,first)
      | else
      |     fprintf('%s -- %s%s- %s Nexteer',NxtrConf,char(169),first,last)
      | end
  DebStepSelection : Subsystem
  HwAg0Snsr0RelCalc : Subsystem
  HwAg0Snsr1RelCalc : Subsystem
  SetNtcSts : Subsystem  RequirementInfo={'linktype_rmi_doors' '0000cf45 (/ESG Group/FDD Module Requirements/EA4 Specific/CM690A_HwAg0Meas)' '#CM690A_71' 'true' 'REQ: CM690A_71' '' } %GIDa_4bb94c51_1b51_4442_a25e_89727b5e18ae
  HwAg0Meas : Outport
  HwAg0TestOk : Outport  Port=2
  wires:
  HwAg0Snsr0Raw/1 -> HwAg0Snsr0RelCalc/1(RawHwAg0Snsr0)
  HwAg0Snsr1Raw/1 -> HwAg0Snsr1RelCalc/1(RawHwAg0Snsr1)
  HwAg0Snsr1RelCalc/1(HwAg0Snsr1Rel) -> AdjStepCalc/2(HwAg0Sns1Rel)
  HwAg0Snsr0RelCalc/1(HwAg0Snsr0Rel) -> AdjStepCalc/1(HwAg0Snsr0Rel)
  AdjStepCalc/1(HwAg0) -> HwAg0Meas/1
  DebStepSelection/1(DebStep) -> SetNtcSts/4(DebStep)
  Constant/1 -> SetNtcSts/1(NtcNr)  "NtcNr"
  AdjStepCalc/2(TestOk) -> DebStepSelection/1(TestOk), SetNtcSts/3(NtcSts), HwAg0TestOk/1
  AdjStepCalc/3(ParamByte) -> SetNtcSts/2(NtcStInfo)

== system CM690A_HwAg0Meas/HwAg0Meas/HwAg0MeasPer4/HwAgRead/If Action Subsystem1 ==
  Action Port : ActionPort  ActionType=then
  CopyRight2 : Subsystem  Description=|  mask(Copyright Information){none=on}
      | Copyright info block.                                               
      |                                                                     
      | Place copyright information at the top of every subsystem in design.
      mask prompts: none "No parameters"
      mask help: Place copyright information at the top of every subsystem in design.
      mask Display:
      | NxtrConf = 'Nexteer Confidential';
      | 
      | sys = bdroot; %handle for the current model ("system")
      | first = get_param(sys,'Created');
      | first = first(end-3:end);  %year is last four digits
      | 
      | last = get_param(sys,'LastModifiedDate');
      | if isempty(last)
      |     last = datestr(now,'yyyy');
      | else
      |     last = last(end-3:end);
      | end
      | 
      | if strcmp(first,last)
      |     fprintf('%s -- Copyright %s Nexteer',NxtrConf,first)
      | else
      |     fprintf('%s -- %s%s- %s Nexteer',NxtrConf,char(169),first,last)
      | end
  Data Type Conversion : DataTypeConversion  OutDataTypeStr=uint8
  SigQlfr : simulink/Sources/Enumerated Constant  OutDataTypeStr=Enum: SigQlfr1  Value=SigQlfr1.SIGQLFR_PASSD  SampleTime=inf
  Qlfr : Outport
  wires:
  SigQlfr/1 -> Data Type Conversion/1
  Data Type Conversion/1 -> Qlfr/1

== system CM690A_HwAg0Meas/HwAg0Meas/HwAg0MeasPer4/HwAgRead/If Action Subsystem2 ==
  note: Information only:
      |
      | - Hold previous value and skip the step
  Action Port : ActionPort  ActionType=else
  CopyRight2 : Subsystem  Description=|  mask(Copyright Information){none=on}
      | Copyright info block.                                               
      |                                                                     
      | Place copyright information at the top of every subsystem in design.
      mask prompts: none "No parameters"
      mask help: Place copyright information at the top of every subsystem in design.
      mask Display:
      | NxtrConf = 'Nexteer Confidential';
      | 
      | sys = bdroot; %handle for the current model ("system")
      | first = get_param(sys,'Created');
      | first = first(end-3:end);  %year is last four digits
      | 
      | last = get_param(sys,'LastModifiedDate');
      | if isempty(last)
      |     last = datestr(now,'yyyy');
      | else
      |     last = last(end-3:end);
      | end
      | 
      | if strcmp(first,last)
      |     fprintf('%s -- Copyright %s Nexteer',NxtrConf,first)
      | else
      |     fprintf('%s -- %s%s- %s Nexteer',NxtrConf,char(169),first,last)
      | end
  Data Type Conversion : DataTypeConversion  OutDataTypeStr=uint8
  NtcSts1 : simulink/Sources/Enumerated Constant  OutDataTypeStr=Enum: NtcSts1  Value=NtcSts1.NTCSTS_PREFAILD  SampleTime=inf
  TestOk : Outport
  wires:
  NtcSts1/1 -> Data Type Conversion/1
  Data Type Conversion/1 -> TestOk/1

== system CM690A_HwAg0Meas/HwAg0Meas/HwAg0MeasPer4/HwAgRead/If Action Subsystem3 ==
  Action Port : ActionPort  ActionType=else
  CopyRight2 : Subsystem  Description=|  mask(Copyright Information){none=on}
      | Copyright info block.                                               
      |                                                                     
      | Place copyright information at the top of every subsystem in design.
      mask prompts: none "No parameters"
      mask help: Place copyright information at the top of every subsystem in design.
      mask Display:
      | NxtrConf = 'Nexteer Confidential';
      | 
      | sys = bdroot; %handle for the current model ("system")
      | first = get_param(sys,'Created');
      | first = first(end-3:end);  %year is last four digits
      | 
      | last = get_param(sys,'LastModifiedDate');
      | if isempty(last)
      |     last = datestr(now,'yyyy');
      | else
      |     last = last(end-3:end);
      | end
      | 
      | if strcmp(first,last)
      |     fprintf('%s -- Copyright %s Nexteer',NxtrConf,first)
      | else
      |     fprintf('%s -- %s%s- %s Nexteer',NxtrConf,char(169),first,last)
      | end
  Data Type Conversion : DataTypeConversion  OutDataTypeStr=uint8
  SigQlfr : simulink/Sources/Enumerated Constant  OutDataTypeStr=Enum: SigQlfr1  Value=SigQlfr1.SIGQLFR_FAILD  SampleTime=inf
  Qlfr : Outport
  wires:
  SigQlfr/1 -> Data Type Conversion/1
  Data Type Conversion/1 -> Qlfr/1

== system CM690A_HwAg0Meas/HwAg0Meas/HwAg0MeasPer5/If Action Subsystem/CopyRight2 ==

== system CM690A_HwAg0Meas/HwAg0Meas/HwAg0MeasPer5/If Action Subsystem1/CopyRight2 ==

== system CM690A_HwAg0Meas/HwAg0Meas/HwAg0MeasPer5/SetNtcSts/CopyRight2 ==

== system CM690A_HwAg0Meas/HwAg0Meas/HwAg0MeasPer2/Snsr0Read/DebStepSelection/CopyRight2 ==

== system CM690A_HwAg0Meas/HwAg0Meas/HwAg0MeasPer2/Snsr0Read/Do nothing/CopyRight2 ==
